simulink model "PID_houseFAST"  (R2024b)
settings: Solver=FixedStepAuto  StartTime=0.0  StopTime=inf  FixedStep=1/f_sim  RelTol=1e-3
model workspace (MATLAB code in the model file):
  | v_max=0.6;      % max |linear speed|
  | max_yaw=1.82;    % max |angular speed|
  | f_sim=1000;      % frequency
values from neighbouring files (symbols this model uses):
  reach_toll = 5*res    [Main_proj2_AstarFAST.m]    (also in Main_proj2_AstarROOMBA.m; Main_proj2_RRT.m = 70*mean(dist))
undefined symbols (not defined in the file or in its folder): Angular, DiscIntNeverNeededParam, Linear, path
libraries: simulink x3, robotlib x3, slpidlib x1
settings Model: Creator=eb  LastModifiedBy=vise
settings OptimizationCC: DefaultParameterBehavior=Inlined  EnhancedBackFolding=on  PassReuseOutputArgsAs=Individual arguments  ZeroExternalMemoryAtStartup=off  ZeroInternalMemoryAtStartup=off  MaxStackSize=64  OptimizeBlockOrder=speed  DifferentSizesBufferReuse=on  OptimizationCustomize=off  EfficientTunableParamExpr=on
settings DebuggingCC: ParameterTunabilityLossMsg=error
settings HardwareCC: ProdBitPerPointer=32  ProdBitPerSizeT=32  ProdBitPerPtrDiffT=32  ProdLargestAtomicFloat=None  ProdIntDivRoundTo=Undefined  ProdEndianess=Unspecified  ProdWordSize=32  ProdHWDeviceType=Generic->Unspecified (assume 32-bit Generic)  UseEmbeddedCoderFeatures=off
settings SFSimCC: MATLABDynamicMemAlloc=off
settings RTWCC: Description=Embedded Coder  SystemTargetFile=ert.tlc  HardwareBoard=Robot Operating System (ROS)  TLCOptions="-aInlineSetEventsForThisBaseRateFcn=TLC_FALSE -aSuppressMultiTaskScheduler=TLC_FALSE  -aRateBasedStepFcn=0"  TemplateMakefile=ert_default_tmf  Toolchain=Catkin  TargetLang=C++
settings CodeAppCC: ForceParamTrailComments=on  IgnoreCustomStorageClasses=off  OperatorAnnotations=on  SimulinkDataObjDesc=on  SFDataObjDesc=on  InsertBlockDesc=on
settings ERTTargetCC: SupportNonInlinedSFcns=on

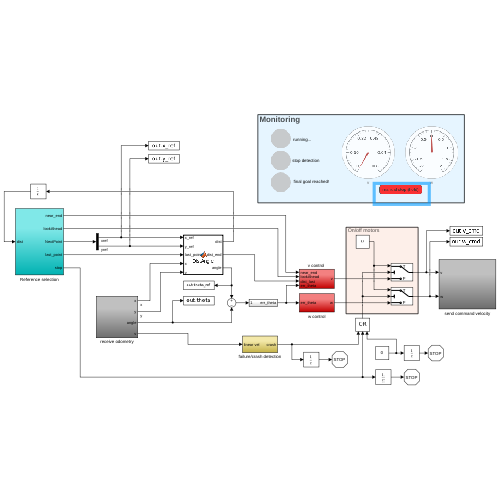
[thumbnail: Simulink's stored preview of the top-level diagram]
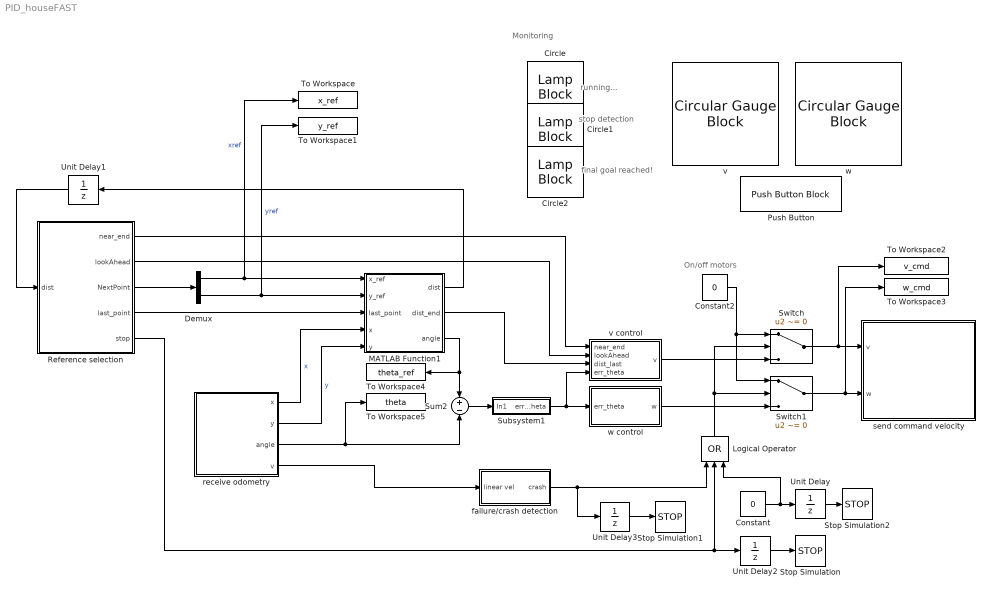
== system PID_houseFAST ==
  note: Monitoring
  note: running...
  note: On/off motors
  note: stop detection
  note: final goal reached!
  Circle : LampBlock  LabelPosition=Hide  Icon=Circle
  Circle1 : LampBlock  LabelPosition=Hide  Icon=Circle
  Circle2 : LampBlock  LabelPosition=Hide  Icon=Circle
  Constant : Constant  Value=0
  Constant2 : Constant  Value=0
  Demux : Demux  Outputs=2
  Logical Operator : Logic  Operator=OR  Inputs=3  AllPortsSameDT=off  OutDataTypeStr=boolean
  MATLAB Function1 : MATLAB Function  TreatAsAtomicUnit=on
  Push Button : PushButtonBlock  ButtonText=manual stop (hold)  IconAlignment=Center  IconColor=On  OffValue=0.000000
  Reference selection : Subsystem
  Stop Simulation : Stop
  Stop Simulation1 : Stop
  Stop Simulation2 : Stop
  Subsystem1 : Subsystem
  Sum2 : Sum  Inputs=+-
  Switch : Switch  Criteria=u2 ~= 0  SaturateOnIntegerOverflow=off  InputSameDT=off
  Switch1 : Switch  Criteria=u2 ~= 0  SaturateOnIntegerOverflow=off  InputSameDT=off
  To Workspace : ToWorkspace  VariableName=x_ref  SampleTime=-1
      settings: Save2DSignal=2-D array (concatenate along first dimension)
  To Workspace1 : ToWorkspace  VariableName=y_ref  SampleTime=-1
      settings: Save2DSignal=2-D array (concatenate along first dimension)
  To Workspace2 : ToWorkspace  VariableName=v_cmd  SampleTime=-1
      settings: Save2DSignal=2-D array (concatenate along first dimension)
  To Workspace3 : ToWorkspace  VariableName=w_cmd  SampleTime=-1
      settings: Save2DSignal=2-D array (concatenate along first dimension)
  To Workspace4 : ToWorkspace  VariableName=theta_ref  SampleTime=-1
      settings: Save2DSignal=2-D array (concatenate along first dimension)
  To Workspace5 : ToWorkspace  VariableName=theta  SampleTime=-1
      settings: Save2DSignal=2-D array (concatenate along first dimension)
  Unit Delay : UnitDelay  SampleTime=0.5  HasFrameUpgradeWarning=on
  Unit Delay1 : UnitDelay  SampleTime=-1  HasFrameUpgradeWarning=on
  Unit Delay2 : UnitDelay  SampleTime=2  HasFrameUpgradeWarning=on
  Unit Delay3 : UnitDelay  SampleTime=0.5  HasFrameUpgradeWarning=on
  failure/crash detection : Subsystem
  receive odometry : Subsystem
  send command velocity : Subsystem
  v : CircularGaugeBlock  LabelPosition=Hide  ScaleMax=0.8
  "v control " : Subsystem
  w : CircularGaugeBlock  LabelPosition=Hide  ScaleMin=-2  ScaleMax=2
  w control : Subsystem
  wires:
  Demux/1 -> To Workspace/1, MATLAB Function1/1(x_ref)  "xref"
  Demux/2 -> To Workspace1/1, MATLAB Function1/2(y_ref)  "yref"
  MATLAB Function1/3(angle) -> To Workspace4/1, Sum2/1
  MATLAB Function1/1(dist) -> Unit Delay1/1
  Sum2/1 -> Subsystem1/1(In1)
  Unit Delay2/1 -> Stop Simulation/1
  Constant2/1 -> Switch1/1, Switch/1
  receive odometry/1(x) -> MATLAB Function1/4(x)  "x"
  receive odometry/2(y) -> MATLAB Function1/5(y)  "y"
  receive odometry/3(angle) -> Sum2/2, To Workspace5/1
  Switch/1 -> To Workspace2/1, send command velocity/1(v)
  Switch1/1 -> To Workspace3/1, send command velocity/2(w)
  Reference selection/5(stop) -> Logical Operator/2, Unit Delay2/1
  Unit Delay1/1 -> Reference selection/1(dist)
  Reference selection/3(NextPoint) -> Demux/1
  receive odometry/4(v) -> failure/crash detection/1(linear vel)
  failure/crash detection/1(crash) -> Unit Delay3/1, Logical Operator/1
  Unit Delay3/1 -> Stop Simulation1/1
  Logical Operator/1 -> Switch1/2, Switch/2
  "v control "/1(v) -> Switch/3
  Subsystem1/1(err_theta) -> "v control "/4(err_theta), w control/1(err_theta)
  w control/1(w) -> Switch1/3
  Reference selection/2(lookAhead) -> "v control "/2(lookAhead)
  Unit Delay/1 -> Stop Simulation2/1
  Constant/1 -> Logical Operator/3, Unit Delay/1
  Reference selection/1(near_end) -> "v control "/1(near_end)
  Reference selection/4(last_point) -> MATLAB Function1/3(last_point)
  MATLAB Function1/2(dist_end) -> "v control "/3(dist_last)

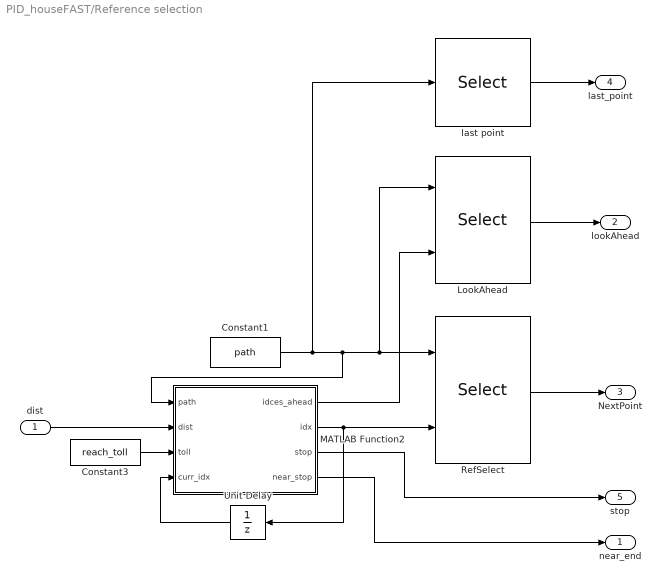
== system PID_houseFAST/Reference selection ==
  dist : Inport
  Constant1 : Constant  Value=path
  Constant3 : Constant  Value=reach_toll
  LookAhead : Selector  NumberOfDimensions=2  IndexOptions=Index vector (port),Select all  Indices=[1 3],[1:2]  OutputSizes=1,1
  MATLAB Function2 : MATLAB Function  TreatAsAtomicUnit=on
  RefSelect : Selector  NumberOfDimensions=2  IndexOptions=Starting index (port),Select all  Indices=[1 3],[1:2]  OutputSizes=1,1
  Unit Delay : UnitDelay  SampleTime=-1  HasFrameUpgradeWarning=on
  last point : Selector  NumberOfDimensions=2  IndexOptions=Index vector (dialog),Select all  Indices=length(path),[1:2]  OutputSizes=1,1
  near_end : Outport
  lookAhead : Outport  Port=2
  NextPoint : Outport  Port=3
  last_point : Outport  Port=4
  stop : Outport  Port=5
  wires:
  MATLAB Function2/1(idces_ahead) -> LookAhead/2
  LookAhead/1 -> lookAhead/1
  MATLAB Function2/2(idx) -> Unit Delay/1, RefSelect/2
  MATLAB Function2/3(stop) -> stop/1
  RefSelect/1 -> NextPoint/1
  Constant1/1 -> last point/1, MATLAB Function2/1(path), LookAhead/1, RefSelect/1
  Unit Delay/1 -> MATLAB Function2/4(curr_idx)
  dist/1 -> MATLAB Function2/2(dist)
  Constant3/1 -> MATLAB Function2/3(toll)
  MATLAB Function2/4(near_stop) -> near_end/1
  last point/1 -> last_point/1

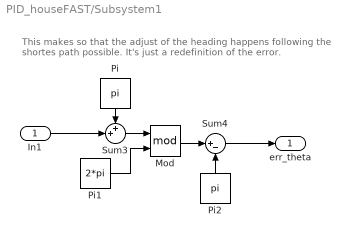
== system PID_houseFAST/Subsystem1 ==
  note: This makes so that the adjust of the heading happens following
      | the shortes path possible. It's just a redefinition of the error.
  In1 : Inport
  Mod : Math  Operator=mod
  Pi : Constant  Value=pi  OutDataTypeStr=Inherit: Inherit via back propagation
  Pi1 : Constant  Value=2*pi  OutDataTypeStr=Inherit: Inherit via back propagation
  Pi2 : Constant  Value=pi  OutDataTypeStr=Inherit: Inherit via back propagation
  Sum3 : Sum  Inputs=++|
  Sum4 : Sum  Inputs=|+-
  err_theta : Outport
  wires:
  Mod/1 -> Sum4/1
  Sum3/1 -> Mod/1
  Pi1/1 -> Mod/2
  Pi/1 -> Sum3/1
  Pi2/1 -> Sum4/2
  In1/1 -> Sum3/2
  Sum4/1 -> err_theta/1

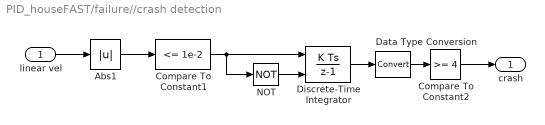
== system PID_houseFAST/failure//crash detection ==
  linear vel : Inport
  Abs1 : Abs  SaturateOnIntegerOverflow=off
  Compare To Constant1 : simulink/Logic and Bit Operations/Compare To Constant  relop=<=  const=1e-2  OutDataTypeStr=boolean
  Compare To Constant2 : simulink/Logic and Bit Operations/Compare To Constant  relop=>=  const=4  OutDataTypeStr=boolean
  Data Type Conversion : DataTypeConversion  SaturateOnIntegerOverflow=off  RndMeth=Floor
  Discrete-Time Integrator : DiscreteIntegrator  ExternalReset=rising  SampleTime=0.1  ICPrevOutput=DiscIntNeverNeededParam  ICPrevScaledInput=DiscIntNeverNeededParam
  NOT : Logic  Operator=NOT  IconShape=distinctive  AllPortsSameDT=off  OutDataTypeStr=boolean
  crash : Outport
  wires:
  linear vel/1 -> Abs1/1
  Abs1/1 -> Compare To Constant1/1
  Compare To Constant1/1 -> NOT/1, Discrete-Time Integrator/1
  Discrete-Time Integrator/1 -> Data Type Conversion/1
  NOT/1 -> Discrete-Time Integrator/2
  Compare To Constant2/1 -> crash/1
  Data Type Conversion/1 -> Compare To Constant2/1

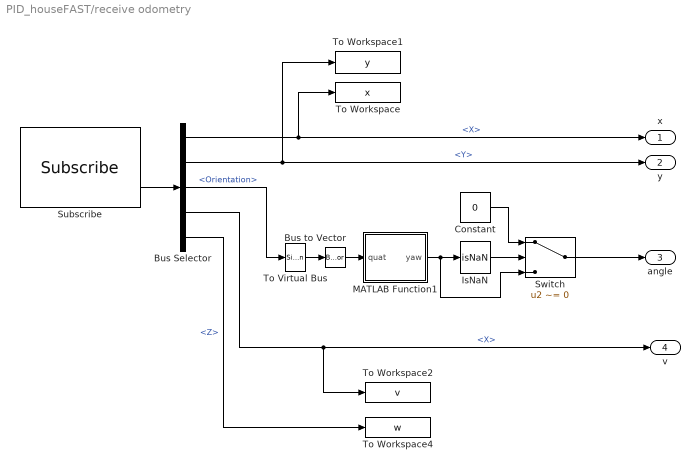
== system PID_houseFAST/receive odometry ==
  Bus Selector : BusSelector  OutputSignals=Pose.Pose.Position.X,Pose.Pose.Position.Y,Pose.Pose.Orientation,Twist.Twist.Linear.X,Twist.Twist.Angular.Z
  Bus to Vector : BusToVector
  Constant : Constant  Value=0
  IsNaN : RelationalOperator  Operator=isNaN  OutDataTypeStr=boolean  RndMeth=Simplest  InputSameDT=off
  MATLAB Function1 : MATLAB Function  TreatAsAtomicUnit=on
  Subscribe : robotlib/Subscribe  topicSource=Select from ROS network  topic=/odom  messageType=nav_msgs/Odometry  SampleTime=1/f_sim  legacyBusStruct=off  messageQueueLength=1
  Switch : Switch  Criteria=u2 ~= 0  SaturateOnIntegerOverflow=off  InputSameDT=off
  To Virtual Bus : SignalConversion  ConversionOutput=Virtual bus  OverrideOpt=off
  To Workspace : ToWorkspace  VariableName=x  SampleTime=-1
      settings: Save2DSignal=2-D array (concatenate along first dimension)
  To Workspace1 : ToWorkspace  VariableName=y  SampleTime=-1
      settings: Save2DSignal=2-D array (concatenate along first dimension)
  To Workspace2 : ToWorkspace  VariableName=v  SampleTime=-1
      settings: Save2DSignal=2-D array (concatenate along first dimension)
  To Workspace4 : ToWorkspace  VariableName=w  SampleTime=-1
      settings: Save2DSignal=2-D array (concatenate along first dimension)
  x : Outport
  y : Outport  Port=2
  angle : Outport  Port=3
  v : Outport  Port=4
  wires:
  Bus Selector/2 -> y/1, To Workspace1/1  "<Y>"
  Subscribe/2 -> Bus Selector/1
  Bus Selector/1 -> x/1, To Workspace/1  "<X>"
  Bus Selector/3 -> To Virtual Bus/1  "<Orientation>"
  Bus to Vector/1 -> MATLAB Function1/1(quat)
  To Virtual Bus/1 -> Bus to Vector/1
  MATLAB Function1/1(yaw) -> IsNaN/1, Switch/3
  IsNaN/1 -> Switch/2
  Constant/1 -> Switch/1
  Bus Selector/4 -> v/1, To Workspace2/1  "<X>"
  Bus Selector/5 -> To Workspace4/1  "<Z>"
  Switch/1 -> angle/1

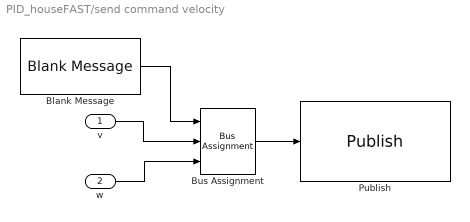
== system PID_houseFAST/send command velocity ==
  v : Inport
  w : Inport  Port=2
  Blank Message : robotlib/Blank Message  messageClass=Message  entityType=geometry_msgs/Twist  messageType=geometry_msgs/Twist  SampleTime=1/f_sim  legacyBusStruct=off
  Bus Assignment : BusAssignment  AssignedSignals=Linear.X,Angular.Z
  Publish : robotlib/Publish  topicSource=Select from ROS network  topic=/cmd_vel  messageType=geometry_msgs/Twist  legacyBusStruct=off  messageQueueLength=1
  wires:
  Blank Message/1 -> Bus Assignment/1
  v/1 -> Bus Assignment/2
  w/1 -> Bus Assignment/3
  Bus Assignment/1 -> Publish/1

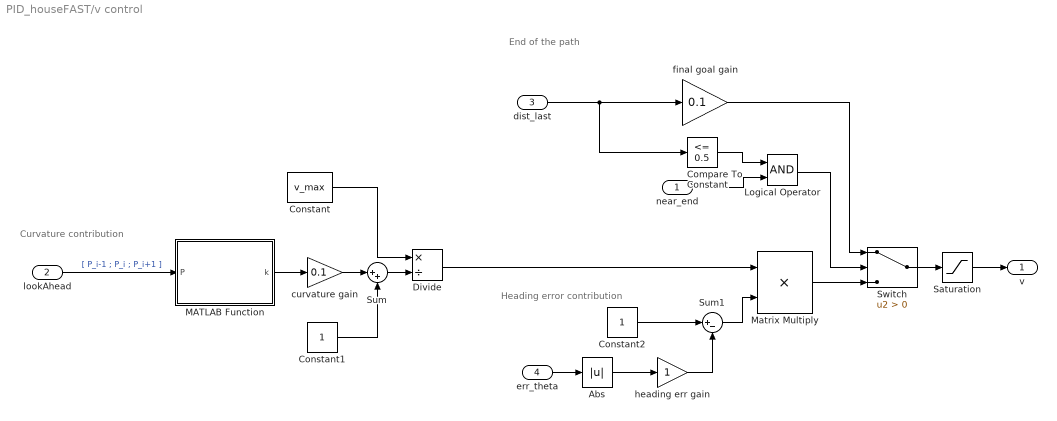
== system PID_houseFAST/v control  ==
  note: Heading error contribution
  note: Curvature contribution
  note: End of the path
  near_end : Inport
  lookAhead : Inport  Port=2
  dist_last : Inport  Port=3
  err_theta : Inport  Port=4
  Abs : Abs  SaturateOnIntegerOverflow=off
  Compare To Constant : simulink/Logic and Bit Operations/Compare To Constant  relop=<=  const=0.5  OutDataTypeStr=boolean
  Constant : Constant  Value=v_max
  Constant1 : Constant
  Constant2 : Constant
  Divide : Product  Inputs=*/
  Logical Operator : Logic  AllPortsSameDT=off  OutDataTypeStr=boolean
  MATLAB Function : MATLAB Function  TreatAsAtomicUnit=on
  Matrix Multiply : Product
  Saturation : Saturate  UpperLimit=v_max  LowerLimit=0
  Sum : Sum  Inputs=|++
  Sum1 : Sum  Inputs=|+-
  Switch : Switch  Criteria=u2 > Threshold  SaturateOnIntegerOverflow=off  InputSameDT=off
  curvature gain : Gain  Gain=0.1
  final goal gain : Gain  Gain=0.1
  heading err gain : Gain
  v : Outport
  wires:
  lookAhead/1 -> MATLAB Function/1(P)  "[ P_i-1 ; P_i ; P_i+1 ]"
  Constant/1 -> Divide/1
  Divide/1 -> Matrix Multiply/1
  Constant1/1 -> Sum/2
  MATLAB Function/1(k) -> curvature gain/1
  curvature gain/1 -> Sum/1
  Sum/1 -> Divide/2
  Matrix Multiply/1 -> Switch/3
  Sum1/1 -> Matrix Multiply/2
  Constant2/1 -> Sum1/1
  err_theta/1 -> Abs/1
  Abs/1 -> heading err gain/1
  heading err gain/1 -> Sum1/2
  Saturation/1 -> v/1
  Switch/1 -> Saturation/1
  final goal gain/1 -> Switch/1
  dist_last/1 -> Compare To Constant/1, final goal gain/1
  Compare To Constant/1 -> Logical Operator/1
  Logical Operator/1 -> Switch/2
  near_end/1 -> Logical Operator/2

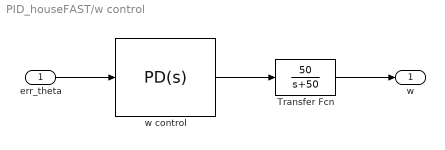
== system PID_houseFAST/w control ==
  err_theta : Inport
  Transfer Fcn : TransferFcn  Numerator=[50]  Denominator=[1 50]
  w control : slpidlib/PID Controller  Controller=PD  Form=Parallel  TimeDomain=Continuous-time  UseExternalTs=off  SampleTime=-1  IntegratorMethod=Forward Euler  FilterMethod=Forward Euler  ControllerParametersSource=internal  P=2.8  I=0.001  UseKiTs=off  D=1  UseExternalDerivativeSource=off  N=15  UseFilter=on  TunerSelectOption=Transfer Function Based (PID Tuner App)  InitialConditionSource=internal  InitialConditionForIntegrator=0  InitialConditionForFilter=0  DifferentiatorICPrevScaledInput=0  ExternalReset=none  TrackingMode=off  Kt=1  LimitOutput=on  SatLimitsSource=internal  UpperSaturationLimit=max_yaw  LowerSaturationLimit=-max_yaw  LinearizeAsGain=on  AntiWindupMode=clamping  Kb=1  LimitIntegrator=off  UpperIntegratorSaturationLimit=inf  LowerIntegratorSaturationLimit=-inf  POutMin=[]  POutMax=[]  IOutMin=[]  IOutMax=[]  DOutMin=[]  DOutMax=[]  NOutMin=[]  NOutMax=[]  SumOutMin=[]  SumOutMax=[]  SaturationOutMin=[]  SaturationOutMax=[]  PParamMin=[]  PParamMax=[]  IParamMin=[]  IParamMax=[]  DParamMin=[]  DParamMax=[]  NParamMin=[]  NParamMax=[]  KbParamMin=[]  KbParamMax=[]  KtParamMin=[]  KtParamMax=[]  KbOutMin=[]  KbOutMax=[]  KtOutMin=[]  KtOutMax=[]  IntegratorOutMin=[]  IntegratorOutMax=[]  FilterOutMin=[]  FilterOutMax=[]  SumI1OutMin=[]  SumI1OutMax=[]  SumI2OutMin=[]  SumI2OutMax=[]  SumI3OutMin=[]  SumI3OutMax=[]  SumI4OutMin=[]  SumI4OutMax=[]  SumDOutMin=[]  SumDOutMax=[]  DifferentiatorOutMin=[]  DifferentiatorOutMax=[]  FilterDiffOutCoefMin=[]  FilterDiffOutCoefMax=[]  ReciprocalOutMin=[]  ReciprocalOutMax=[]  SumDenOutMin=[]  SumDenOutMax=[]  SumNumOutMin=[]  SumNumOutMax=[]  DivideOutMin=[]  DivideOutMax=[]  UdiffTsProdOutMin=[]  UdiffTsProdOutMax=[]  NTsProdOutMin=[]  NTsProdOutMax=[]  UintegralTsProdOutMin=[]  UintegralTsProdOutMax=[]  UngainTsProdOutMin=[]  UngainTsProdOutMax=[]  ClampingZeroOutDataTypeStr=Inherit: Inherit via back propagation  ClampingZeroOutMin=[]  ClampingZeroOutMax=[]  FilterDenConstantOutDataTypeStr=Inherit: Inherit via back propagation  FilterDenConstantOutMin=[]  FilterDenConstantOutMax=[]  PCopyOutDataTypeStr=Inherit: Inherit via back propagation  PCopyOutMin=[]  PCopyOutMax=[]  NCopyOutDataTypeStr=Inherit: Inherit via back propagation  NCopyOutMin=[]  NCopyOutMax=[]  IntegratorContinuousStateAttributes=''  IntegratorStateMustResolveToSignalObject=off  IntegratorRTWStateStorageClass=Auto  FilterContinuousStateAttributes=''  FilterStateMustResolveToSignalObject=off  FilterRTWStateStorageClass=Auto  ParallelPVariant=InternalParameters  IdealPVariant=Disabled  IVariant=Disabled  DVariant=InternalParameters  IntegratorVariant=Disabled  SatVariant=Enabled  AWVariant=Disabled  PCopyVariant=Disabled  TRVariant=Disabled  FdbkBlocksVariant=Forward  IdealPFdbkVariant=Disabled  SatFdbkVariant=Disabled  DerivativeFilterVariant=ContFilter  NVariant=InternalParameters  NCopyVariant=Disabled  FilterICVariant=InternalICsFilter  IntegratorICVariant=Disabled  ExternalResetVariant=Disabled  TRSumVariant=Passthrough  SumFdbkVariant=Disabled  SumVariant=Sum_PD  TsampFilterVariant=InternalTs  TsampNgainVariant=Passthrough  TsampIntegralVariant=Disabled_SignalSpec  ExternalSaturationOutDataTypeStr=Inherit: Same as second input  DerivativeSourceVariant=ErrorSignal  PreIntVariant=InternalPreInt
  w : Outport
  wires:
  err_theta/1 -> w control/1
  w control/1 -> Transfer Fcn/1
  Transfer Fcn/1 -> w/1

== matlab function PID_houseFAST/MATLAB Function1 ==
  data: x_ref input; y_ref input; last_point input; x input; dist output; dist_end output; angle output; y input
function [dist,dist_end,angle]=DistAngle(x_ref,y_ref,last_point,x,y)

% Distance and orientation wrt the next reference point
delta_x=x_ref-x;
delta_y=y_ref-y;
dist=sqrt(delta_x.^2+delta_y.^2);
angle=atan2(delta_y,delta_x);

% Distance wrt the last point
x_end=last_point(1);
y_end=last_point(2);
dist_end=sqrt((x_end-x).^2+(y_end-y).^2);

end

== matlab function PID_houseFAST/v control /MATLAB Function ==
  data: P input; k output
function k=Curvature(P)

% Extract 3 future points coordinates
x1=P(1,1);
x2=P(2,1);
x3=P(3,1);
y1=P(1,2);
y2=P(2,2);
y3=P(3,2);

% Curvature
k=abs((x3-x2)*(y2-y1)-(x2-x1)*(y3-y2))/abs((x3-x2)^2+(y3-y2)^2)^(3/2);

end

== matlab function PID_houseFAST/Reference selection/MATLAB Function2 ==
  data: idces_ahead output; idx output; stop output; near_stop output; path input; dist input; toll input; curr_idx input
function [idces_ahead,idx,stop,near_stop]=RefIdxSelect(path,dist,toll,curr_idx)

% For heading control 
stop=false;
near_stop=false;
N_max=length(path);
if curr_idx<N_max && curr_idx>0
    if dist<toll
        idx=min(curr_idx+3,N_max);
    else
        idx=curr_idx;
    end
elseif curr_idx==0
    idx=1;
else 
    idx=N_max;
    if dist<toll
        stop=true;
    end
end

% For linear velocity control (turns)
idces_ahead=idx+[5 6 7];
if idces_ahead(end)>N_max
    idces_ahead=[N_max-2 N_max-1 N_max];
end

% For slowing down before endpoint
if curr_idx>=N_max-150
    near_stop=true;
end

end

== matlab function PID_houseFAST/receive odometry/MATLAB Function1 ==
  data: quat input; yaw output
function yaw=quat2yaw(quat)

q=zeros(1,4);

q(1)=quat(1);
q(2)=quat(2);
q(3)=quat(3);
q(4)=quat(4);

eul=quat2eul(q);

yaw=eul(3);

end
